simulink model "MIL4L3_SW6_V1_20220211"  (R2018b)
settings: Solver=FixedStepAuto  StartTime=0.0  StopTime=inf  FixedStep=0.001  RelTol=1e-3
PreLoadFcn:
  | A0_MILtest;
undefined symbols (not defined in the file or in its folder): Clb_ICADirect_LaneDisp_StateFive, Clb_ICADirect_LaneDisp_StateFour, Clb_ICADirect_LaneDisp_StateOne, Clb_ICADirect_LaneDisp_StateThree, Clb_ICADirect_LaneDisp_StateTwo, Clb_ICADirect_LaneDisp_StateZero, Clb_ICADirect_LaneDispSW, Clb_ICADirect_TrnLghtsCom_Switch, Clb_ICADirect_TrnLghtsCom_Value, Clb_ICADirect_TrnLghtsCrtl_Inhb, IMAP_Clb_ACU_Driver_Belt, IMAP_Clb_ACU_Driver_Belt_Over, IMAP_Clb_ACU_Passenger_Belt, IMAP_Clb_ACU_Passenger_Belt_Over, IMAP_Clb_ACU_RearLeft_Belt, IMAP_Clb_ACU_RearLeft_Belt_Over, IMAP_Clb_ACU_RearMiddle_Belt, IMAP_Clb_ACU_RearMiddle_Belt_Over, IMAP_Clb_ACU_RearRight_Belt, IMAP_Clb_ACU_RearRight_Belt_Over, IMAP_Clb_AEB_Switch, IMAP_Clb_AEB_Switch_Over, IMAP_Clb_ALC_TLC_Mode, IMAP_Clb_ALC_TLC_Mode_Over, IMAP_Clb_BCM_Battery_Voltage, IMAP_Clb_BCM_Battery_Voltage_Over, IMAP_Clb_BCM_BrakeLamp_State, IMAP_Clb_BCM_BrakeLamp_State_Over, IMAP_Clb_BCM_CHMSL_Status, IMAP_Clb_BCM_CHMSL_Status_Over, IMAP_Clb_BCM_Door_Lock_State, IMAP_Clb_BCM_Door_Lock_State_Over, IMAP_Clb_BCM_FrontWiper_State, IMAP_Clb_BCM_FrontWiper_State_Over, IMAP_Clb_BCM_FrontWiper_Switch, IMAP_Clb_BCM_FrontWiper_Switch_Over, IMAP_Clb_BCM_HazardLamp, IMAP_Clb_BCM_HazardLamp_Over, IMAP_Clb_BCM_HazardLamp_Switch, IMAP_Clb_BCM_HazardLamp_Switch_Over, IMAP_Clb_BCM_HighBeam_State, IMAP_Clb_BCM_HighBeam_State_Over, IMAP_Clb_BCM_Ignition_State, IMAP_Clb_BCM_Ignition_State_Over, IMAP_Clb_BCM_IHBC_Enabled, IMAP_Clb_BCM_IHBC_Enabled_Over, IMAP_Clb_BCM_Left_Light, IMAP_Clb_BCM_Left_Light_Over, IMAP_Clb_BCM_LeftTurn_Switch, IMAP_Clb_BCM_LeftTurn_Switch_Over, IMAP_Clb_BCM_LF_Door_State, IMAP_Clb_BCM_LF_Door_State_Over, IMAP_Clb_BCM_LowBeam_State, IMAP_Clb_BCM_LowBeam_State_Over, IMAP_Clb_BCM_LR_Door_State, IMAP_Clb_BCM_LR_Door_State_Over, IMAP_Clb_BCM_RF_Door_State, IMAP_Clb_BCM_RF_Door_State_Over, IMAP_Clb_BCM_Right_Light, IMAP_Clb_BCM_Right_Light_Over ... (+547)
libraries: CarMaker4SL x2153, simulink x292, dspstat3 x3, canmsglib x2, simulink_extras x1
(part 27 of 52)

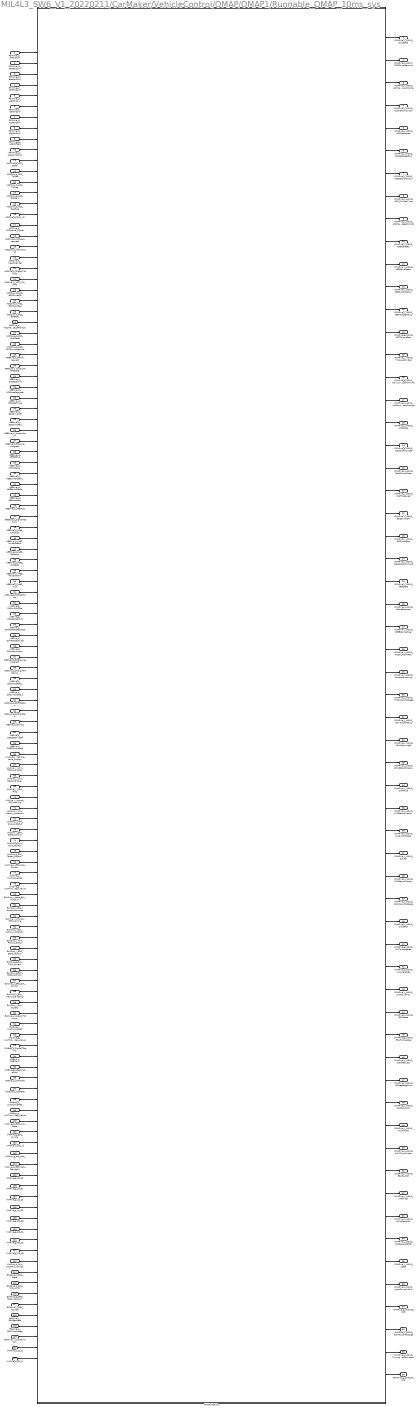
== system MIL4L3_SW6_V1_20220211/CarMaker/VehicleControl/OMAP/OMAP1/Runnable_OMAP_10ms_sys ==
  FDMMve_d_JaFcnConf : Inport  OutDataTypeStr=uint16  PortDimensions=1
  FDMMve_d_AebFcnConf : Inport  Port=2  OutDataTypeStr=uint16  PortDimensions=1
  FDMMve_d_EsaFcnConf : Inport  Port=3  OutDataTypeStr=uint16  PortDimensions=1
  FDMMve_d_ElkFcnConf : Inport  Port=4  OutDataTypeStr=uint16  PortDimensions=1
  FDMMve_d_LkaFcnConf : Inport  Port=5  OutDataTypeStr=uint16  PortDimensions=1
  FDMMve_d_IcaFcnConf : Inport  Port=6  OutDataTypeStr=uint16  PortDimensions=1
  FDMMve_d_AccFcnConf : Inport  Port=7  OutDataTypeStr=uint16  PortDimensions=1
  FDMMve_d_EwFcnConf : Inport  Port=8  OutDataTypeStr=uint16  PortDimensions=1
  FDMMve_g_Adas2Fapa : Inport  Port=9  OutDataTypeStr=uint32  PortDimensions=1
  FDMMve_d_SignalTStamp : Inport  Port=10  OutDataTypeStr=uint16  PortDimensions=1
  ACCSve_d_ACC_State : Inport  Port=11  OutDataTypeStr=uint16  PortDimensions=1
  ACCSve_g_ACC_TqReq : Inport  Port=12  OutDataTypeStr=single  PortDimensions=1
  ACCSve_d_ACC_TqFlag : Inport  Port=13  OutDataTypeStr=uint16  PortDimensions=1
  ACCSve_g_ACC_DecReq : Inport  Port=14  OutDataTypeStr=single  PortDimensions=1
  ACCSve_d_ACC_DecFlag : Inport  Port=15  OutDataTypeStr=uint16  PortDimensions=1
  ACCSve_d_CIPV_ID : Inport  Port=16  OutDataTypeStr=uint16  PortDimensions=1
  ACCSve_d_ACCActive_Signal : Inport  Port=17  OutDataTypeStr=uint16  PortDimensions=1
  ACCSve_d_ACC_go_request : Inport  Port=18  OutDataTypeStr=uint16  PortDimensions=1
  ACCSve_d_VelocitySet : Inport  Port=19  OutDataTypeStr=uint16  PortDimensions=1
  ACCSve_d_HeadWaySet : Inport  Port=20  OutDataTypeStr=uint16  PortDimensions=1
  ACCSve_d_SignalTStamp : Inport  Port=21  OutDataTypeStr=uint16  PortDimensions=1
  ACCSve_d_ACC_ICA_Flag : Inport  Port=22  OutDataTypeStr=uint16  PortDimensions=1
  ACCSve_d_ACC_ESCDriveOff : Inport  Port=23  OutDataTypeStr=uint16  PortDimensions=1
  ACCSve_d_ACC_ESCHoldReq : Inport  Port=24  OutDataTypeStr=uint16  PortDimensions=1
  ACCSve_d_ACC_EPBReq : Inport  Port=25  OutDataTypeStr=uint16  PortDimensions=1
  ACCSve_d_ACCMessagePrompt : Inport  Port=26  OutDataTypeStr=uint16
  ACCSve_d_ACC_ISLCState : Inport  Port=27  OutDataTypeStr=uint16  PortDimensions=1
  ACCSve_d_ACC_ISLCDriverRemind : Inport  Port=28  OutDataTypeStr=uint16  PortDimensions=1
  AEBSve_d_Prefill_request : Inport  Port=29  OutDataTypeStr=uint16  PortDimensions=1
  AEBSve_d_functionFARCState : Inport  Port=30  OutDataTypeStr=uint16  PortDimensions=1
  AEBSve_g_DecSetpoint : Inport  Port=31  OutDataTypeStr=single  PortDimensions=1
  AEBSve_d_MDDdecRequest : Inport  Port=32  OutDataTypeStr=uint16  PortDimensions=1
  AEBSve_d_MDDdecType : Inport  Port=33  OutDataTypeStr=uint16  PortDimensions=1
  AEBSve_d_ESCDriveOff : Inport  Port=34  OutDataTypeStr=uint16  PortDimensions=1
  AEBSve_d_ESCHoldReq : Inport  Port=35  OutDataTypeStr=uint16  PortDimensions=1
  AEBSve_d_HapticAlarm : Inport  Port=36  OutDataTypeStr=uint16  PortDimensions=1
  AEBSve_d_Braking_progress : Inport  Port=37  OutDataTypeStr=uint16  PortDimensions=1
  AEBSve_d_AEBStatus : Inport  Port=38  OutDataTypeStr=uint16  PortDimensions=1
  AEBSve_d_FCWStatus : Inport  Port=39  OutDataTypeStr=uint16  PortDimensions=1
  AEBSve_d_AEBSwitchStatus : Inport  Port=40  OutDataTypeStr=uint16  PortDimensions=1
  AEBSve_d_AEBFaultStatus : Inport  Port=41  OutDataTypeStr=uint16  PortDimensions=1
  AEBSve_d_AEBAlertReq : Inport  Port=42  OutDataTypeStr=uint16  PortDimensions=1
  AEBSve_d_AEBTips : Inport  Port=43  OutDataTypeStr=uint16  PortDimensions=1
  AEBSve_d_SignalTStamp : Inport  Port=44  OutDataTypeStr=uint16  PortDimensions=1
  AEBSve_d_JABS_AlertSign : Inport  Port=45  OutDataTypeStr=uint16  PortDimensions=1
  AEBSve_d_JABS_SwitchStatus : Inport  Port=46  OutDataTypeStr=uint16  PortDimensions=1
  AEBSve_d_JABS_FltStatus : Inport  Port=47  OutDataTypeStr=uint16  PortDimensions=1
  AEBSve_d_JABS_AlertReq : Inport  Port=48  OutDataTypeStr=uint16  PortDimensions=1
  AEBSve_d_JABS_HapticAlarm : Inport  Port=49  OutDataTypeStr=uint16  PortDimensions=1
  AEBSve_d_JABS_Tips : Inport  Port=50  OutDataTypeStr=uint16  PortDimensions=1
  JABSve_d_DbPrefillReq : Inport  Port=51  OutDataTypeStr=uint16  PortDimensions=1
  JABSve_d_DbFunFARCSta : Inport  Port=52  OutDataTypeStr=uint16  PortDimensions=1
  JABSve_g_DbDecSetpoint : Inport  Port=53  OutDataTypeStr=single  PortDimensions=1
  JABSve_d_DbMDDdecRequest : Inport  Port=54  OutDataTypeStr=uint16  PortDimensions=1
  JABSve_d_DbMDDdecType : Inport  Port=55  OutDataTypeStr=uint16  PortDimensions=1
  JABSve_d_DbHapticAlarm : Inport  Port=56  OutDataTypeStr=uint16  PortDimensions=1
  JABSve_d_DbBraking_progress : Inport  Port=57  OutDataTypeStr=uint16  PortDimensions=1
  JABSve_d_DbSignalTStamp : Inport  Port=58  OutDataTypeStr=uint16  PortDimensions=1
  JABSve_d_DbJACWStatus : Inport  Port=59  OutDataTypeStr=uint16  PortDimensions=1
  JABSve_d_DbSwitchStatus : Inport  Port=60  OutDataTypeStr=uint16  PortDimensions=1
  JABSve_d_DbFltStatus : Inport  Port=61  OutDataTypeStr=uint16  PortDimensions=1
  JABSve_d_DbAlertReq : Inport  Port=62  OutDataTypeStr=uint16  PortDimensions=1
  JABSve_d_DbTips : Inport  Port=63  OutDataTypeStr=uint16  PortDimensions=1
  JABSve_d_DbESCDriveOff : Inport  Port=64  OutDataTypeStr=uint16  PortDimensions=1
  JABSve_d_DbESCHoldReq : Inport  Port=65  OutDataTypeStr=uint16  PortDimensions=1
  LKASve_y_Vehicle_Lane_Display : Inport  Port=66  OutDataTypeStr=uint8  PortDimensions=1
  LKASve_y_LDW_Status_Display : Inport  Port=67  OutDataTypeStr=uint8  PortDimensions=1
  LKASve_y_LKA_Status_Display : Inport  Port=68  OutDataTypeStr=uint8  PortDimensions=1
  LKASve_y_LDW_Flag : Inport  Port=69  OutDataTypeStr=uint8  PortDimensions=1
  LKASve_y_Hands_Off_Warning : Inport  Port=70  OutDataTypeStr=uint8  PortDimensions=1
  LKASve_y_LKA_Action_Indication : Inport  Port=71  OutDataTypeStr=uint8  PortDimensions=1
  LKASve_y_HMI_Popup_Status : Inport  Port=72  OutDataTypeStr=uint8  PortDimensions=1
  LKASve_y_EPS_State_Control : Inport  Port=73  OutDataTypeStr=uint8  PortDimensions=1
  LKASve_g_LKA_SWA_Control : Inport  Port=74  OutDataTypeStr=single  PortDimensions=1
  LKASve_g_EPS_Factor_Control : Inport  Port=75  OutDataTypeStr=single  PortDimensions=1
  LKASve_y_EPS_LKA_Control : Inport  Port=76  OutDataTypeStr=uint8  PortDimensions=1
  LKASve_y_LKATorqueReq : Inport  Port=77  OutDataTypeStr=uint8  PortDimensions=1
  LKASve_g_LKATorqueReq_Value : Inport  Port=78  OutDataTypeStr=single  PortDimensions=1
  ELKSve_y_state_ELK_function : Inport  Port=79  OutDataTypeStr=uint8  PortDimensions=1
  ELKSve_y_ELK_HapticAlarmReq : Inport  Port=80  OutDataTypeStr=uint8  PortDimensions=1
  ELKSve_y_Hands_Off_Warning : Inport  Port=81  OutDataTypeStr=uint8  PortDimensions=1
  ELKSve_y_ELK_Action_Indication : Inport  Port=82  OutDataTypeStr=uint8  PortDimensions=1
  ELKSve_y_HMI_Popup_Status : Inport  Port=83  OutDataTypeStr=uint8  PortDimensions=1
  ELKSve_y_EPS_State_Control : Inport  Port=84  OutDataTypeStr=uint8  PortDimensions=1
  ELKSve_g_ELK_SWA_Control : Inport  Port=85  OutDataTypeStr=single  PortDimensions=1
  ELKSve_g_EPS_Factor_Control : Inport  Port=86  OutDataTypeStr=single  PortDimensions=1
  ELKSve_y_EPS_ELK_Control : Inport  Port=87  OutDataTypeStr=uint8  PortDimensions=1
  ELKSve_y_ELK_VehicleLaneDisp : Inport  Port=88  OutDataTypeStr=uint8  PortDimensions=1
  ELKSve_y_ELK_ELKSts : Inport  Port=89  OutDataTypeStr=uint8  PortDimensions=1
  ELKSve_y_SignalTStamp : Inport  Port=90  OutDataTypeStr=uint8  PortDimensions=1
  ELKSve_y_LKATorqueReq : Inport  Port=91  OutDataTypeStr=uint8  PortDimensions=1
  ELKSve_g_LKATorqueReq_Value : Inport  Port=92  OutDataTypeStr=single  PortDimensions=1
  ICABve_d_SignalTStamp : Inport  Port=93  OutDataTypeStr=uint16  PortDimensions=1
  ICABva_d_ICAB2HMI : Inport  Port=94  OutDataTypeStr=uint16  PortDimensions=20
  ICABve_g_SteerAngleCmd : Inport  Port=95  OutDataTypeStr=single  PortDimensions=1
  ICABve_d_ICAMode : Inport  Port=96  OutDataTypeStr=uint16  PortDimensions=1
  ICABve_d_ICAState : Inport  Port=97  OutDataTypeStr=uint16  PortDimensions=1
  ICABve_d_LKATorqueReq : Inport  Port=98  OutDataTypeStr=uint16  PortDimensions=1
  ICABve_g_LKATorqueReq_Value : Inport  Port=99  OutDataTypeStr=single  PortDimensions=1
  IMAPve_d_EPS_LKA_State : Inport  Port=100  OutDataTypeStr=uint16  PortDimensions=1
  IMAPve_g_ESC_LonAcc : Inport  Port=101  OutDataTypeStr=single  PortDimensions=1
  IMAPva_d_obj_id : Inport  Port=102  OutDataTypeStr=uint16  PortDimensions=40
  IMAPva_g_obj_pos_x : Inport  Port=103  OutDataTypeStr=single  PortDimensions=40
  IMAPve_d_ESC_Veh_Standstill : Inport  Port=104  OutDataTypeStr=uint16  PortDimensions=1
  IMAPve_g_L0_C0 : Inport  Port=105  OutDataTypeStr=single  PortDimensions=1
  IMAPve_g_L0_C1 : Inport  Port=106  OutDataTypeStr=single  PortDimensions=1
  IMAPve_g_L0_C2 : Inport  Port=107  OutDataTypeStr=single  PortDimensions=1
  IMAPve_g_L0_C3 : Inport  Port=108  OutDataTypeStr=single  PortDimensions=1
  IMAPve_g_R0_C0 : Inport  Port=109  OutDataTypeStr=single  PortDimensions=1
  IMAPve_g_R0_C1 : Inport  Port=110  OutDataTypeStr=single  PortDimensions=1
  IMAPve_g_R0_C2 : Inport  Port=111  OutDataTypeStr=single  PortDimensions=1
  IMAPve_g_R0_C3 : Inport  Port=112  OutDataTypeStr=single  PortDimensions=1
  IMAPve_d_APA_AutoPark_WorkSt : Inport  Port=113  OutDataTypeStr=uint16  PortDimensions=1
  ESASve_y_ESA_State : Inport  Port=114  OutDataTypeStr=uint8
  ESASve_g_ESA_SWA_CMD : Inport  Port=115  OutDataTypeStr=single
  ESASve_g_EPS_Factor_Control : Inport  Port=116  OutDataTypeStr=single
  ESASve_y_ESA_FaultSt : Inport  Port=117  OutDataTypeStr=uint8
  ESASve_y_ESARequest : Inport  Port=118  OutDataTypeStr=uint8
  ESASve_y_ESATorqueReq : Inport  Port=119  OutDataTypeStr=single
  ESASve_y_LKAActivation : Inport  Port=120  OutDataTypeStr=uint8
  IMAPve_d_L0_Q : Inport  Port=121  OutDataTypeStr=uint16
  IMAPve_d_R0_Q : Inport  Port=122  OutDataTypeStr=uint16
  OMAP_Module : Subsystem  TreatAsAtomicUnit=on
  OMAPve_y_ADAS_ISLCState : Outport  OutDataTypeStr=uint8  PortDimensions=1
  OMAPve_y_ADAS_ISLCDriverRemind : Outport  Port=2  OutDataTypeStr=uint8  PortDimensions=1
  OMAPve_y_ADAS_ACCHeadwayDisplay : Outport  Port=3  OutDataTypeStr=uint8  PortDimensions=1
  OMAPve_y_ADAS_ACCHeadwayIcon : Outport  Port=4  OutDataTypeStr=uint8  PortDimensions=1
  OMAPve_y_ADAS_ACCSetSpeed : Outport  Port=5  OutDataTypeStr=uint8  PortDimensions=1
  OMAPve_y_ADAS_ACCSetSpeedDis : Outport  Port=6  OutDataTypeStr=uint8  PortDimensions=1
  OMAPve_y_ADAS_ACCStatusIconDis : Outport  Port=7  OutDataTypeStr=uint8  PortDimensions=1
  OMAPve_y_ADAS_ACC_RVVReqType : Outport  Port=8  OutDataTypeStr=uint8  PortDimensions=1
  OMAPve_y_ADAS_ACCMessagePrompt : Outport  Port=9  OutDataTypeStr=uint8  PortDimensions=1
  OMAPve_y_ADAS_AEBAlertReq : Outport  Port=10  OutDataTypeStr=uint8  PortDimensions=1
  OMAPve_y_ADAS_AEBFaultStatus : Outport  Port=11  OutDataTypeStr=uint8  PortDimensions=1
  OMAPve_y_ADAS_AEBSwitchStatus : Outport  Port=12  OutDataTypeStr=uint8  PortDimensions=1
  OMAPve_y_ADAS_AEBMassageDisp : Outport  Port=13  OutDataTypeStr=uint8  PortDimensions=1
  OMAPve_g_ADAS_ACCTorqueReq : Outport  Port=14  OutDataTypeStr=single  PortDimensions=1
  OMAPve_y_ADAS_TorqueActivReq : Outport  Port=15  OutDataTypeStr=uint8  PortDimensions=1
  OMAPve_g_ADAS_DownorUpGearMinTime : Outport  Port=16  OutDataTypeStr=single  PortDimensions=1
  OMAPve_y_ADAS_UpDownGearChange : Outport  Port=17  OutDataTypeStr=uint8  PortDimensions=1
  OMAPve_y_ADAS_ACCState : Outport  Port=18  OutDataTypeStr=uint8  PortDimensions=1
  OMAPve_g_ADAS_DecelerationSet : Outport  Port=19  OutDataTypeStr=single  PortDimensions=1
  OMAPve_y_ADAS_DeclControlReq : Outport  Port=20  OutDataTypeStr=uint8  PortDimensions=1
  OMAPve_y_ADAS_PrefillRequest : Outport  Port=21  OutDataTypeStr=uint8  PortDimensions=1
  OMAPve_y_ADAS_ESCDriveOff : Outport  Port=22  OutDataTypeStr=uint8  PortDimensions=1
  OMAPve_y_ADAS_ESCHoldReq : Outport  Port=23  OutDataTypeStr=uint8  PortDimensions=1
  OMAPve_y_ADAS_DecelerationType : Outport  Port=24  OutDataTypeStr=uint8  PortDimensions=1
  OMAPve_y_ADAS_AEBState : Outport  Port=25  OutDataTypeStr=uint8  PortDimensions=1
  OMAPve_y_ADAS_BrakeRequest : Outport  Port=26  OutDataTypeStr=uint8  PortDimensions=1
  OMAPve_y_ADAS_AEBBrakingProg : Outport  Port=27  OutDataTypeStr=uint8  PortDimensions=1
  OMAPve_y_ADAS_HapticAlarmReq : Outport  Port=28  OutDataTypeStr=uint8  PortDimensions=1
  OMAPve_y_ADAS_Handsoffwarning : Outport  Port=29  OutDataTypeStr=uint8  PortDimensions=1
  OMAPve_y_ADAS_HMIPopupMassage : Outport  Port=30  OutDataTypeStr=uint8  PortDimensions=1
  OMAPve_y_ADAS_VehicleLaneDisp : Outport  Port=31  OutDataTypeStr=uint8  PortDimensions=1
  OMAPve_y_ADAS_LDWWarningSt : Outport  Port=32  OutDataTypeStr=uint8  PortDimensions=1
  OMAPve_y_ADAS_LDWStatusDisplay : Outport  Port=33  OutDataTypeStr=uint8  PortDimensions=1
  OMAPve_y_ADAS_LKAMode : Outport  Port=34  OutDataTypeStr=uint8  PortDimensions=1
  OMAPve_y_ADAS_LKAStatusDisplay : Outport  Port=35  OutDataTypeStr=uint8  PortDimensions=1
  OMAPve_y_ADAS_LKASwitchState : Outport  Port=36  OutDataTypeStr=uint8  PortDimensions=1
  OMAPve_y_ADAS_ELKSts : Outport  Port=37  OutDataTypeStr=uint8  PortDimensions=1
  OMAPve_y_ADAS_LCAStatusDisplay : Outport  Port=38  OutDataTypeStr=uint8  PortDimensions=1
  OMAPve_y_ADAS_LCAPopupMessage : Outport  Port=39  OutDataTypeStr=uint8  PortDimensions=1
  OMAPve_y_ADAS_LKAState : Outport  Port=40  OutDataTypeStr=uint8  PortDimensions=1
  OMAPve_g_ADAS_LKATorqFactReq : Outport  Port=41  OutDataTypeStr=single  PortDimensions=1
  OMAPve_g_ADAS_LKAAngleReq : Outport  Port=42  OutDataTypeStr=single  PortDimensions=1
  OMAPve_y_ADAS_LKAActivation : Outport  Port=43  OutDataTypeStr=uint8  PortDimensions=1
  OMAPve_y_ADAS_ESAState : Outport  Port=44  OutDataTypeStr=uint8  PortDimensions=1
  OMAPve_g_ADAS_ESATorqueReq : Outport  Port=45  OutDataTypeStr=single  PortDimensions=1
  OMAPve_y_ADAS_ESARequest : Outport  Port=46  OutDataTypeStr=uint8  PortDimensions=1
  OMAPve_y_ADAS_ICAMassageDisp : Outport  Port=47  OutDataTypeStr=uint8  PortDimensions=1
  OMAPve_y_ADAS_ICAStatusIcon : Outport  Port=48  OutDataTypeStr=uint8  PortDimensions=1
  OMAPve_y_ADAS_HWAMode : Outport  Port=49  OutDataTypeStr=uint8  PortDimensions=1
  OMAPve_y_ADAS_HWATurnOnIdctr : Outport  Port=50  OutDataTypeStr=uint8  PortDimensions=1
  OMAPve_y_ADAS_ESAFaultSt : Outport  Port=51  OutDataTypeStr=uint8  PortDimensions=1
  OMAPve_y_ADAS_JAFaultSt : Outport  Port=52  OutDataTypeStr=uint8  PortDimensions=1
  OMAPve_y_ADAS_HWAActionSts : Outport  Port=53  OutDataTypeStr=uint8  PortDimensions=1
  OMAPve_y_ADAS_ACCRequestEPB : Outport  Port=54  OutDataTypeStr=uint8  PortDimensions=1
  OMAPve_y_ADAS_State : Outport  Port=55  OutDataTypeStr=uint8  PortDimensions=1
  OMAPve_y_ADAS_LightControlValid : Outport  Port=56  OutDataTypeStr=uint8  PortDimensions=1
  OMAPve_g_ob019L_100 : Outport  Port=57  OutDataTypeStr=uint32  PortDimensions=1
  OMAPve_y_ADAS_ELKPopupMessage : Outport  Port=58  OutDataTypeStr=uint8
  OMAPve_y_ADAS_TurnLightsCommand : Outport  Port=59  OutDataTypeStr=uint8
  FDMMve_g_ob019H_100 : Outport  Port=60  OutDataTypeStr=uint32
  wires:
  ELKSve_y_HMI_Popup_Status/1 -> OMAP_Module/83(ELKSve_y_HMI_Popup_Status)
  FDMMve_d_ElkFcnConf/1 -> OMAP_Module/4(FDMMve_d_ElkFcnConf)
  AEBSve_d_AEBFaultStatus/1 -> OMAP_Module/41(AEBSve_d_AEBFaultStatus)
  OMAP_Module/36(OMAPve_y_ADAS_LKASwitchState) -> OMAPve_y_ADAS_LKASwitchState/1
  AEBSve_d_Braking_progress/1 -> OMAP_Module/37(AEBSve_d_Braking_progress)
  OMAP_Module/9(OMAPve_y_ADAS_ACCMessagePrompt) -> OMAPve_y_ADAS_ACCMessagePrompt/1
  OMAP_Module/31(OMAPve_y_ADAS_VehicleLaneDisp) -> OMAPve_y_ADAS_VehicleLaneDisp/1
  FDMMve_d_AebFcnConf/1 -> OMAP_Module/2(FDMMve_d_AebFcnConf)
  ACCSve_d_ACC_DecFlag/1 -> OMAP_Module/15(ACCSve_d_ACC_DecFlag)
  ICABva_d_ICAB2HMI/1 -> OMAP_Module/94(ICABva_d_ICAB2HMI)
  OMAP_Module/32(OMAPve_y_ADAS_LDWWarningSt) -> OMAPve_y_ADAS_LDWWarningSt/1
  AEBSve_d_AEBStatus/1 -> OMAP_Module/38(AEBSve_d_AEBStatus)
  IMAPve_d_ESC_Veh_Standstill/1 -> OMAP_Module/104(IMAPve_d_ESC_Veh_Standstill)
  FDMMve_g_Adas2Fapa/1 -> OMAP_Module/9(FDMMve_g_Adas2Fapa)
  OMAP_Module/41(OMAPve_g_ADAS_LKATorqFactReq) -> OMAPve_g_ADAS_LKATorqFactReq/1
  ELKSve_g_ELK_SWA_Control/1 -> OMAP_Module/85(ELKSve_g_ELK_SWA_Control)
  FDMMve_d_IcaFcnConf/1 -> OMAP_Module/6(FDMMve_d_IcaFcnConf)
  LKASve_y_EPS_State_Control/1 -> OMAP_Module/73(LKASve_y_EPS_State_Control)
  OMAP_Module/14(OMAPve_g_ADAS_ACCTorqueReq) -> OMAPve_g_ADAS_ACCTorqueReq/1
  ELKSve_y_ELK_ELKSts/1 -> OMAP_Module/89(ELKSve_y_ELK_ELKSts)
  ICABve_d_SignalTStamp/1 -> OMAP_Module/93(ICABve_d_SignalTStamp)
  AEBSve_d_MDDdecRequest/1 -> OMAP_Module/32(AEBSve_d_MDDdecRequest)
  ELKSve_y_state_ELK_function/1 -> OMAP_Module/79(ELKSve_y_state_ELK_function)
  OMAP_Module/6(OMAPve_y_ADAS_ACCSetSpeedDis) -> OMAPve_y_ADAS_ACCSetSpeedDis/1
  ACCSve_d_ACCActive_Signal/1 -> OMAP_Module/17(ACCSve_d_ACCActive_Signal)
  AEBSve_g_DecSetpoint/1 -> OMAP_Module/31(AEBSve_g_DecSetpoint)
  IMAPve_g_L0_C2/1 -> OMAP_Module/107(IMAPve_g_L0_C2)
  JABSve_d_DbSwitchStatus/1 -> OMAP_Module/60(JABSve_d_DbSwitchStatus)
  ACCSve_d_VelocitySet/1 -> OMAP_Module/19(ACCSve_d_VelocitySet)
  ELKSve_y_SignalTStamp/1 -> OMAP_Module/90(ELKSve_y_SignalTStamp)
  ACCSve_d_ACC_ICA_Flag/1 -> OMAP_Module/22(ACCSve_d_ACC_ICA_Flag)
  AEBSve_d_AEBAlertReq/1 -> OMAP_Module/42(AEBSve_d_AEBAlertReq)
  JABSve_d_DbMDDdecType/1 -> OMAP_Module/55(JABSve_d_DbMDDdecType)
  OMAP_Module/13(OMAPve_y_ADAS_AEBMassageDisp) -> OMAPve_y_ADAS_AEBMassageDisp/1
  LKASve_y_EPS_LKA_Control/1 -> OMAP_Module/76(LKASve_y_EPS_LKA_Control)
  ELKSve_y_ELK_Action_Indication/1 -> OMAP_Module/82(ELKSve_y_ELK_Action_Indication)
  AEBSve_d_JABS_FltStatus/1 -> OMAP_Module/47(AEBSve_d_JABS_FltStatus)
  OMAP_Module/47(OMAPve_y_ADAS_ICAMassageDisp) -> OMAPve_y_ADAS_ICAMassageDisp/1
  OMAP_Module/4(OMAPve_y_ADAS_ACCHeadwayIcon) -> OMAPve_y_ADAS_ACCHeadwayIcon/1
  OMAP_Module/8(OMAPve_y_ADAS_ACC_RVVReqType) -> OMAPve_y_ADAS_ACC_RVVReqType/1
  JABSve_d_DbPrefillReq/1 -> OMAP_Module/51(JABSve_d_DbPrefillReq)
  LKASve_y_LDW_Status_Display/1 -> OMAP_Module/67(LKASve_y_LDW_Status_Display)
  AEBSve_d_JABS_Tips/1 -> OMAP_Module/50(AEBSve_d_JABS_Tips)
  AEBSve_d_JABS_AlertReq/1 -> OMAP_Module/48(AEBSve_d_JABS_AlertReq)
  AEBSve_d_JABS_AlertSign/1 -> OMAP_Module/45(AEBSve_d_JABS_AlertSign)
  OMAP_Module/11(OMAPve_y_ADAS_AEBFaultStatus) -> OMAPve_y_ADAS_AEBFaultStatus/1
  AEBSve_d_FCWStatus/1 -> OMAP_Module/39(AEBSve_d_FCWStatus)
  JABSve_d_DbFunFARCSta/1 -> OMAP_Module/52(JABSve_d_DbFunFARCSta)
  AEBSve_d_SignalTStamp/1 -> OMAP_Module/44(AEBSve_d_SignalTStamp)
  ELKSve_g_EPS_Factor_Control/1 -> OMAP_Module/86(ELKSve_g_EPS_Factor_Control)
  IMAPve_g_R0_C1/1 -> OMAP_Module/110(IMAPve_g_R0_C1)
  JABSve_d_DbTips/1 -> OMAP_Module/63(JABSve_d_DbTips)
  AEBSve_d_functionFARCState/1 -> OMAP_Module/30(AEBSve_d_functionFARCState)
  JABSve_d_DbBraking_progress/1 -> OMAP_Module/57(JABSve_d_DbBraking_progress)
  AEBSve_d_MDDdecType/1 -> OMAP_Module/33(AEBSve_d_MDDdecType)
  LKASve_y_Vehicle_Lane_Display/1 -> OMAP_Module/66(LKASve_y_Vehicle_Lane_Display)
  AEBSve_d_HapticAlarm/1 -> OMAP_Module/36(AEBSve_d_HapticAlarm)
  OMAP_Module/12(OMAPve_y_ADAS_AEBSwitchStatus) -> OMAPve_y_ADAS_AEBSwitchStatus/1
  OMAP_Module/5(OMAPve_y_ADAS_ACCSetSpeed) -> OMAPve_y_ADAS_ACCSetSpeed/1
  ELKSve_y_EPS_State_Control/1 -> OMAP_Module/84(ELKSve_y_EPS_State_Control)
  OMAP_Module/26(OMAPve_y_ADAS_BrakeRequest) -> OMAPve_y_ADAS_BrakeRequest/1
  AEBSve_d_ESCHoldReq/1 -> OMAP_Module/35(AEBSve_d_ESCHoldReq)
  OMAP_Module/21(OMAPve_y_ADAS_PrefillRequest) -> OMAPve_y_ADAS_PrefillRequest/1
  OMAP_Module/43(OMAPve_y_ADAS_LKAActivation) -> OMAPve_y_ADAS_LKAActivation/1
  ACCSve_g_ACC_DecReq/1 -> OMAP_Module/14(ACCSve_g_ACC_DecReq)
  ACCSve_g_ACC_TqReq/1 -> OMAP_Module/12(ACCSve_g_ACC_TqReq)
  OMAP_Module/10(OMAPve_y_ADAS_AEBAlertReq) -> OMAPve_y_ADAS_AEBAlertReq/1
  OMAP_Module/50(OMAPve_y_ADAS_HWATurnOnIdctr) -> OMAPve_y_ADAS_HWATurnOnIdctr/1
  JABSve_d_DbSignalTStamp/1 -> OMAP_Module/58(JABSve_d_DbSignalTStamp)
  ELKSve_y_EPS_ELK_Control/1 -> OMAP_Module/87(ELKSve_y_EPS_ELK_Control)
  IMAPve_g_L0_C0/1 -> OMAP_Module/105(IMAPve_g_L0_C0)
  IMAPva_d_obj_id/1 -> OMAP_Module/102(IMAPva_d_obj_id)
  OMAP_Module/2(OMAPve_y_ADAS_ISLCDriverRemind) -> OMAPve_y_ADAS_ISLCDriverRemind/1
  JABSve_d_DbHapticAlarm/1 -> OMAP_Module/56(JABSve_d_DbHapticAlarm)
  AEBSve_d_AEBTips/1 -> OMAP_Module/43(AEBSve_d_AEBTips)
  IMAPve_g_R0_C3/1 -> OMAP_Module/112(IMAPve_g_R0_C3)
  ACCSve_d_CIPV_ID/1 -> OMAP_Module/16(ACCSve_d_CIPV_ID)
  OMAP_Module/27(OMAPve_y_ADAS_AEBBrakingProg) -> OMAPve_y_ADAS_AEBBrakingProg/1
  LKASve_y_LKA_Action_Indication/1 -> OMAP_Module/71(LKASve_y_LKA_Action_Indication)
  OMAP_Module/3(OMAPve_y_ADAS_ACCHeadwayDisplay) -> OMAPve_y_ADAS_ACCHeadwayDisplay/1
  ACCSve_d_ACC_go_request/1 -> OMAP_Module/18(ACCSve_d_ACC_go_request)
  IMAPve_g_L0_C1/1 -> OMAP_Module/106(IMAPve_g_L0_C1)
  LKASve_g_EPS_Factor_Control/1 -> OMAP_Module/75(LKASve_g_EPS_Factor_Control)
  OMAP_Module/22(OMAPve_y_ADAS_ESCDriveOff) -> OMAPve_y_ADAS_ESCDriveOff/1
  JABSve_d_DbMDDdecRequest/1 -> OMAP_Module/54(JABSve_d_DbMDDdecRequest)
  OMAP_Module/38(OMAPve_y_ADAS_LCAStatusDisplay) -> OMAPve_y_ADAS_LCAStatusDisplay/1
  OMAP_Module/28(OMAPve_y_ADAS_HapticAlarmReq) -> OMAPve_y_ADAS_HapticAlarmReq/1
  FDMMve_d_AccFcnConf/1 -> OMAP_Module/7(FDMMve_d_AccFcnConf)
  JABSve_d_DbESCHoldReq/1 -> OMAP_Module/65(JABSve_d_DbESCHoldReq)
  OMAP_Module/25(OMAPve_y_ADAS_AEBState) -> OMAPve_y_ADAS_AEBState/1
  OMAP_Module/16(OMAPve_g_ADAS_DownorUpGearMinTime) -> OMAPve_g_ADAS_DownorUpGearMinTime/1
  OMAP_Module/20(OMAPve_y_ADAS_DeclControlReq) -> OMAPve_y_ADAS_DeclControlReq/1
  OMAP_Module/29(OMAPve_y_ADAS_Handsoffwarning) -> OMAPve_y_ADAS_Handsoffwarning/1
  OMAP_Module/53(OMAPve_y_ADAS_HWAActionSts) -> OMAPve_y_ADAS_HWAActionSts/1
  OMAP_Module/15(OMAPve_y_ADAS_TorqueActivReq) -> OMAPve_y_ADAS_TorqueActivReq/1
  OMAP_Module/30(OMAPve_y_ADAS_HMIPopupMassage) -> OMAPve_y_ADAS_HMIPopupMassage/1
  IMAPve_g_ESC_LonAcc/1 -> OMAP_Module/101(IMAPve_g_ESC_LonAcc)
  AEBSve_d_Prefill_request/1 -> OMAP_Module/29(AEBSve_d_Prefill_request)
  ACCSve_d_ACC_ESCDriveOff/1 -> OMAP_Module/23(ACCSve_d_ACC_ESCDriveOff)
  IMAPve_g_R0_C0/1 -> OMAP_Module/109(IMAPve_g_R0_C0)
  OMAP_Module/34(OMAPve_y_ADAS_LKAMode) -> OMAPve_y_ADAS_LKAMode/1
  OMAP_Module/44(OMAPve_y_ADAS_ESAState) -> OMAPve_y_ADAS_ESAState/1
  OMAP_Module/33(OMAPve_y_ADAS_LDWStatusDisplay) -> OMAPve_y_ADAS_LDWStatusDisplay/1
  LKASve_y_LDW_Flag/1 -> OMAP_Module/69(LKASve_y_LDW_Flag)
  ELKSve_y_ELK_VehicleLaneDisp/1 -> OMAP_Module/88(ELKSve_y_ELK_VehicleLaneDisp)
  OMAP_Module/18(OMAPve_y_ADAS_ACCState) -> OMAPve_y_ADAS_ACCState/1
  OMAP_Module/52(OMAPve_y_ADAS_JAFaultSt) -> OMAPve_y_ADAS_JAFaultSt/1
  JABSve_d_DbFltStatus/1 -> OMAP_Module/61(JABSve_d_DbFltStatus)
  OMAP_Module/56(OMAPve_y_ADAS_LightControlValid) -> OMAPve_y_ADAS_LightControlValid/1
  ACCSve_d_ACC_ESCHoldReq/1 -> OMAP_Module/24(ACCSve_d_ACC_ESCHoldReq)
  OMAP_Module/54(OMAPve_y_ADAS_ACCRequestEPB) -> OMAPve_y_ADAS_ACCRequestEPB/1
  OMAP_Module/37(OMAPve_y_ADAS_ELKSts) -> OMAPve_y_ADAS_ELKSts/1
  LKASve_y_HMI_Popup_Status/1 -> OMAP_Module/72(LKASve_y_HMI_Popup_Status)
  OMAP_Module/7(OMAPve_y_ADAS_ACCStatusIconDis) -> OMAPve_y_ADAS_ACCStatusIconDis/1
  FDMMve_d_EwFcnConf/1 -> OMAP_Module/8(FDMMve_d_EwFcnConf)
  JABSve_d_DbJACWStatus/1 -> OMAP_Module/59(JABSve_d_DbJACWStatus)
  JABSve_g_DbDecSetpoint/1 -> OMAP_Module/53(JABSve_g_DbDecSetpoint)
  ICABve_d_ICAMode/1 -> OMAP_Module/96(ICABve_d_ICAMode)
  LKASve_y_Hands_Off_Warning/1 -> OMAP_Module/70(LKASve_y_Hands_Off_Warning)
  LKASve_y_LKA_Status_Display/1 -> OMAP_Module/68(LKASve_y_LKA_Status_Display)
  JABSve_d_DbAlertReq/1 -> OMAP_Module/62(JABSve_d_DbAlertReq)
  OMAP_Module/42(OMAPve_g_ADAS_LKAAngleReq) -> OMAPve_g_ADAS_LKAAngleReq/1
  OMAP_Module/40(OMAPve_y_ADAS_LKAState) -> OMAPve_y_ADAS_LKAState/1
  OMAP_Module/23(OMAPve_y_ADAS_ESCHoldReq) -> OMAPve_y_ADAS_ESCHoldReq/1
  AEBSve_d_JABS_HapticAlarm/1 -> OMAP_Module/49(AEBSve_d_JABS_HapticAlarm)
  OMAP_Module/45(OMAPve_g_ADAS_ESATorqueReq) -> OMAPve_g_ADAS_ESATorqueReq/1
  OMAP_Module/48(OMAPve_y_ADAS_ICAStatusIcon) -> OMAPve_y_ADAS_ICAStatusIcon/1
  OMAP_Module/17(OMAPve_y_ADAS_UpDownGearChange) -> OMAPve_y_ADAS_UpDownGearChange/1
  IMAPve_d_EPS_LKA_State/1 -> OMAP_Module/100(IMAPve_d_EPS_LKA_State)
  ACCSve_d_ACC_TqFlag/1 -> OMAP_Module/13(ACCSve_d_ACC_TqFlag)
  OMAP_Module/49(OMAPve_y_ADAS_HWAMode) -> OMAPve_y_ADAS_HWAMode/1
  FDMMve_d_EsaFcnConf/1 -> OMAP_Module/3(FDMMve_d_EsaFcnConf)
  IMAPve_g_R0_C2/1 -> OMAP_Module/111(IMAPve_g_R0_C2)
  OMAP_Module/24(OMAPve_y_ADAS_DecelerationType) -> OMAPve_y_ADAS_DecelerationType/1
  ACCSve_d_ACC_EPBReq/1 -> OMAP_Module/25(ACCSve_d_ACC_EPBReq)
  OMAP_Module/19(OMAPve_g_ADAS_DecelerationSet) -> OMAPve_g_ADAS_DecelerationSet/1
  AEBSve_d_AEBSwitchStatus/1 -> OMAP_Module/40(AEBSve_d_AEBSwitchStatus)
  JABSve_d_DbESCDriveOff/1 -> OMAP_Module/64(JABSve_d_DbESCDriveOff)
  OMAP_Module/35(OMAPve_y_ADAS_LKAStatusDisplay) -> OMAPve_y_ADAS_LKAStatusDisplay/1
  AEBSve_d_JABS_SwitchStatus/1 -> OMAP_Module/46(AEBSve_d_JABS_SwitchStatus)
  OMAP_Module/55(OMAPve_y_ADAS_State) -> OMAPve_y_ADAS_State/1
  OMAP_Module/51(OMAPve_y_ADAS_ESAFaultSt) -> OMAPve_y_ADAS_ESAFaultSt/1
  IMAPva_g_obj_pos_x/1 -> OMAP_Module/103(IMAPva_g_obj_pos_x)
  OMAP_Module/1(OMAPve_y_ADAS_ISLCState) -> OMAPve_y_ADAS_ISLCState/1
  ACCSve_d_SignalTStamp/1 -> OMAP_Module/21(ACCSve_d_SignalTStamp)
  FDMMve_d_LkaFcnConf/1 -> OMAP_Module/5(FDMMve_d_LkaFcnConf)
  OMAP_Module/46(OMAPve_y_ADAS_ESARequest) -> OMAPve_y_ADAS_ESARequest/1
  OMAP_Module/39(OMAPve_y_ADAS_LCAPopupMessage) -> OMAPve_y_ADAS_LCAPopupMessage/1
  ICABve_d_ICAState/1 -> OMAP_Module/97(ICABve_d_ICAState)
  ELKSve_y_Hands_Off_Warning/1 -> OMAP_Module/81(ELKSve_y_Hands_Off_Warning)
  AEBSve_d_ESCDriveOff/1 -> OMAP_Module/34(AEBSve_d_ESCDriveOff)
  ELKSve_y_ELK_HapticAlarmReq/1 -> OMAP_Module/80(ELKSve_y_ELK_HapticAlarmReq)
  ACCSve_d_HeadWaySet/1 -> OMAP_Module/20(ACCSve_d_HeadWaySet)
  LKASve_g_LKA_SWA_Control/1 -> OMAP_Module/74(LKASve_g_LKA_SWA_Control)
  ICABve_g_SteerAngleCmd/1 -> OMAP_Module/95(ICABve_g_SteerAngleCmd)
  IMAPve_g_L0_C3/1 -> OMAP_Module/108(IMAPve_g_L0_C3)
  FDMMve_d_JaFcnConf/1 -> OMAP_Module/1(FDMMve_d_JaFcnConf)
  FDMMve_d_SignalTStamp/1 -> OMAP_Module/10(FDMMve_d_SignalTStamp)
  ACCSve_d_ACC_State/1 -> OMAP_Module/11(ACCSve_d_ACC_State)
  LKASve_y_LKATorqueReq/1 -> OMAP_Module/77(LKASve_y_LKATorqueReq)
  LKASve_g_LKATorqueReq_Value/1 -> OMAP_Module/78(LKASve_g_LKATorqueReq_Value)
  ELKSve_y_LKATorqueReq/1 -> OMAP_Module/91(ELKSve_y_LKATorqueReq)
  ELKSve_g_LKATorqueReq_Value/1 -> OMAP_Module/92(ELKSve_g_LKATorqueReq_Value)
  ICABve_d_LKATorqueReq/1 -> OMAP_Module/98(ICABve_d_LKATorqueReq)
  ICABve_g_LKATorqueReq_Value/1 -> OMAP_Module/99(ICABve_g_LKATorqueReq_Value)
  IMAPve_d_APA_AutoPark_WorkSt/1 -> OMAP_Module/113(IMAPve_d_APA_AutoPark_WorkSt)
  OMAP_Module/57(OMAPve_g_ob019L_100) -> OMAPve_g_ob019L_100/1
  ACCSve_d_ACC_ISLCState/1 -> OMAP_Module/27(ACCSve_d_ACC_ISLCState)
  ACCSve_d_ACC_ISLCDriverRemind/1 -> OMAP_Module/28(ACCSve_d_ACC_ISLCDriverRemind)
  OMAP_Module/58(OMAPve_y_ADAS_ELKPopupMessage) -> OMAPve_y_ADAS_ELKPopupMessage/1
  OMAP_Module/59(OMAPve_y_ADAS_TurnLightsCommand) -> OMAPve_y_ADAS_TurnLightsCommand/1
  ESASve_y_ESA_State/1 -> OMAP_Module/114(ESASve_y_ESA_State)
  ESASve_g_ESA_SWA_CMD/1 -> OMAP_Module/115(ESASve_g_ESA_SWA_CMD)
  ESASve_g_EPS_Factor_Control/1 -> OMAP_Module/116(ESASve_g_EPS_Factor_Control)
  ESASve_y_ESA_FaultSt/1 -> OMAP_Module/117(ESASve_y_ESA_FaultSt)
  ESASve_y_ESARequest/1 -> OMAP_Module/118(ESASve_y_ESARequest)
  ESASve_y_ESATorqueReq/1 -> OMAP_Module/119(ESASve_y_ESATorqueReq)
  ESASve_y_LKAActivation/1 -> OMAP_Module/120(ESASve_y_LKAActivation)
  ACCSve_d_ACCMessagePrompt/1 -> OMAP_Module/26(ACCSve_d_ACCMessagePrompt)
  OMAP_Module/60(FDMMve_g_ob019H_100) -> FDMMve_g_ob019H_100/1
  IMAPve_d_L0_Q/1 -> OMAP_Module/121(IMAPve_d_L0_Q)
  IMAPve_d_R0_Q/1 -> OMAP_Module/122(IMAPve_d_R0_Q)

== system MIL4L3_SW6_V1_20220211/CarMaker/VehicleControl/SDFADataLog/Subsystem40/Subsystem ==
  Compare To Constant : simulink/Logic and Bit Operations/Compare To Constant  relop=>=  const=1  OutDataTypeStr=boolean
  Compare To Constant1 : simulink/Logic and Bit Operations/Compare To Constant  relop=>  const=0  OutDataTypeStr=boolean
  Const tar_id5 : Constant  Value=0
  Data Type Conversion : DataTypeConversion
  Digital Clock : DigitalClock  SampleTime=0.06
  Logical Operator : Logic  AllPortsSameDT=off  OutDataTypeStr=boolean
  Read CM Dict1 : CarMaker4SL/Read CM Dict  xname=Sensor.Object.Radar.relvTgt.dtct  xsync=off
  Read CM Dict7 : CarMaker4SL/Read CM Dict  xname=User.IO.Out.NumberOfObj  xsync=off
  Switch15 : Switch  Criteria=u2 > Threshold
  Radar_timestamp : Outport
  wires:
  Logical Operator/1 -> Switch15/2  "<dtct>"
  Digital Clock/1 -> Data Type Conversion/1
  Data Type Conversion/1 -> Switch15/1
  Switch15/1 -> Radar_timestamp/1  "Radar_timestamp"
  Const tar_id5/1 -> Switch15/3
  Read CM Dict7/1 -> Compare To Constant/1
  Compare To Constant/1 -> Logical Operator/2
  Read CM Dict1/1 -> Compare To Constant1/1
  Compare To Constant1/1 -> Logical Operator/1

== system MIL4L3_SW6_V1_20220211/CarMaker/VehicleControl/SDFADataLog/Subsystem40/Subsystem1 ==
  Compare To Constant : simulink/Logic and Bit Operations/Compare To Constant  relop=>=  const=2  OutDataTypeStr=boolean
  Compare To Constant1 : simulink/Logic and Bit Operations/Compare To Constant  relop=>  const=0  OutDataTypeStr=boolean
  Const tar_id5 : Constant  Value=0
  Data Type Conversion : DataTypeConversion
  Digital Clock : DigitalClock  SampleTime=0.06
  Logical Operator : Logic  AllPortsSameDT=off  OutDataTypeStr=boolean
  Read CM Dict1 : CarMaker4SL/Read CM Dict  xname=Sensor.Object.Radar.relvTgt.dtct  xsync=off
  Read CM Dict7 : CarMaker4SL/Read CM Dict  xname=User.IO.Out.NumberOfObj  xsync=off
  Switch15 : Switch  Criteria=u2 > Threshold
  Radar_timestamp : Outport
  wires:
  Compare To Constant1/1 -> Logical Operator/1
  Read CM Dict1/1 -> Compare To Constant1/1
  Compare To Constant/1 -> Logical Operator/2
  Read CM Dict7/1 -> Compare To Constant/1
  Const tar_id5/1 -> Switch15/3
  Switch15/1 -> Radar_timestamp/1  "Radar_timestamp"
  Data Type Conversion/1 -> Switch15/1
  Digital Clock/1 -> Data Type Conversion/1
  Logical Operator/1 -> Switch15/2  "<dtct>"

== system MIL4L3_SW6_V1_20220211/CarMaker/VehicleControl/SDFADataLog/Subsystem40/Subsystem2 ==
  Compare To Constant : simulink/Logic and Bit Operations/Compare To Constant  relop=>=  const=3  OutDataTypeStr=boolean
  Compare To Constant1 : simulink/Logic and Bit Operations/Compare To Constant  relop=>  const=0  OutDataTypeStr=boolean
  Const tar_id5 : Constant  Value=0
  Data Type Conversion : DataTypeConversion
  Digital Clock : DigitalClock  SampleTime=0.06
  Logical Operator : Logic  AllPortsSameDT=off  OutDataTypeStr=boolean
  Read CM Dict1 : CarMaker4SL/Read CM Dict  xname=Sensor.Object.Radar.relvTgt.dtct  xsync=off
  Read CM Dict7 : CarMaker4SL/Read CM Dict  xname=User.IO.Out.NumberOfObj  xsync=off
  Switch15 : Switch  Criteria=u2 > Threshold
  Radar_timestamp : Outport
  wires:
  Logical Operator/1 -> Switch15/2  "<dtct>"
  Digital Clock/1 -> Data Type Conversion/1
  Data Type Conversion/1 -> Switch15/1
  Switch15/1 -> Radar_timestamp/1  "Radar_timestamp"
  Const tar_id5/1 -> Switch15/3
  Read CM Dict7/1 -> Compare To Constant/1
  Compare To Constant/1 -> Logical Operator/2
  Read CM Dict1/1 -> Compare To Constant1/1
  Compare To Constant1/1 -> Logical Operator/1

== system MIL4L3_SW6_V1_20220211/CarMaker/VehicleControl/SDFADataLog/Subsystem40/Subsystem3 ==
  Compare To Constant : simulink/Logic and Bit Operations/Compare To Constant  relop=>=  const=4  OutDataTypeStr=boolean
  Compare To Constant1 : simulink/Logic and Bit Operations/Compare To Constant  relop=>  const=0  OutDataTypeStr=boolean
  Const tar_id5 : Constant  Value=0
  Data Type Conversion : DataTypeConversion
  Digital Clock : DigitalClock  SampleTime=0.06
  Logical Operator : Logic  AllPortsSameDT=off  OutDataTypeStr=boolean
  Read CM Dict1 : CarMaker4SL/Read CM Dict  xname=Sensor.Object.Radar.relvTgt.dtct  xsync=off
  Read CM Dict7 : CarMaker4SL/Read CM Dict  xname=User.IO.Out.NumberOfObj  xsync=off
  Switch15 : Switch  Criteria=u2 > Threshold
  Radar_timestamp : Outport
  wires:
  Compare To Constant1/1 -> Logical Operator/1
  Read CM Dict1/1 -> Compare To Constant1/1
  Compare To Constant/1 -> Logical Operator/2
  Read CM Dict7/1 -> Compare To Constant/1
  Const tar_id5/1 -> Switch15/3
  Switch15/1 -> Radar_timestamp/1  "Radar_timestamp"
  Data Type Conversion/1 -> Switch15/1
  Digital Clock/1 -> Data Type Conversion/1
  Logical Operator/1 -> Switch15/2  "<dtct>"

== system MIL4L3_SW6_V1_20220211/CarMaker/VehicleControl/SwitchForRealECU_ACC_Gas/PI Control/Subsystem1 ==
  -1 : Constant
  -2 : Constant
  -3 : Constant  Value=13.515
  -4 : Constant
  0 : Constant
  1 : Constant  Value=15.604
  2 : Constant  Value=11.1
  3 : Constant  Value=6.986
  4 : Constant  Value=4.737
  5 : Constant  Value=3.311
  6 : Constant  Value=2.356
  Multiport Switch : MultiPortSwitch  DataPortOrder=Specify indices  Inputs=9  DataPortIndices={0,1,2,3,4,5,6,7,8,-1}  DataPortForDefault=Additional data port
  Read CM Dict20 : CarMaker4SL/Read CM Dict  xname=PT.GearBox.GearNo  xsync=off
  TCU_AGB_position : Outport
  wires:
  -4/1 -> Multiport Switch/12
  -3/1 -> Multiport Switch/11
  Multiport Switch/1 -> TCU_AGB_position/1  "TCU_AGB_position"
  -2/1 -> Multiport Switch/10
  6/1 -> Multiport Switch/8
  1/1 -> Multiport Switch/3
  5/1 -> Multiport Switch/7
  2/1 -> Multiport Switch/4
  0/1 -> Multiport Switch/2
  -1/1 -> Multiport Switch/9
  4/1 -> Multiport Switch/6
  3/1 -> Multiport Switch/5
  Read CM Dict20/1 -> Multiport Switch/1

== system MIL4L3_SW6_V1_20220211/CarMaker/IPG Vehicle/CarAndTrailer/Forces/Tires/TireFL ==
  note: Insert your tire model here.
  Sync_In : Inport
  Load : Inport  Port=2
  vxtrans : Inport  Port=3
  vytrans : Inport  Port=4
  Rim_rotv : Inport  Port=5
  Rim_turnv : Inport  Port=6
  InclinAngle : Inport  Port=7
  muRoad : Inport  Port=8
  Ground{1..11} (11 alike) : Ground
  Terminator{,1..6,12} (8 alike) : Terminator
  Slp : Outport
  Alpha : Outport  Port=2
  TurnSlp : Outport  Port=3
  rBelt_eff : Outport  Port=4
  vBelt : Outport  Port=5
  LongFrc : Outport  Port=6
  SideFrc : Outport  Port=7
  LoadFrc : Outport  Port=8
  OverturnTrq : Outport  Port=9
  RollResist : Outport  Port=10
  AlignTrq : Outport  Port=11
  wires:
  Ground11/1 -> vBelt/1
  Ground10/1 -> rBelt_eff/1
  Ground9/1 -> TurnSlp/1
  Rim_turnv/1 -> Terminator6/1
  Sync_In/1 -> Terminator12/1
  Ground2/1 -> Alpha/1
  Ground3/1 -> LongFrc/1
  Ground4/1 -> SideFrc/1
  Ground5/1 -> OverturnTrq/1
  vxtrans/1 -> Terminator1/1
  vytrans/1 -> Terminator2/1
  Rim_rotv/1 -> Terminator3/1
  InclinAngle/1 -> Terminator4/1
  muRoad/1 -> Terminator5/1
  Load/1 -> Terminator/1
  Ground1/1 -> Slp/1
  Ground6/1 -> LoadFrc/1
  Ground7/1 -> RollResist/1
  Ground8/1 -> AlignTrq/1

== system MIL4L3_SW6_V1_20220211/CarMaker/IPG Vehicle/CarAndTrailer/Forces/Tires/TireFR ==
  note: Insert your tire model here.
  Sync_In : Inport
  Load : Inport  Port=2
  vxtrans : Inport  Port=3
  vytrans : Inport  Port=4
  Rim_rotv : Inport  Port=5
  Rim_turnv : Inport  Port=6
  InclinAngle : Inport  Port=7
  muRoad : Inport  Port=8
  Ground{1..11} (11 alike) : Ground
  Terminator{,1..6,12} (8 alike) : Terminator
  Slp : Outport
  Alpha : Outport  Port=2
  TurnSlp : Outport  Port=3
  rBelt_eff : Outport  Port=4
  vBelt : Outport  Port=5
  LongFrc : Outport  Port=6
  SideFrc : Outport  Port=7
  LoadFrc : Outport  Port=8
  OverturnTrq : Outport  Port=9
  RollResist : Outport  Port=10
  AlignTrq : Outport  Port=11
  wires:
  Ground11/1 -> vBelt/1
  Ground10/1 -> rBelt_eff/1
  Ground9/1 -> TurnSlp/1
  Rim_turnv/1 -> Terminator6/1
  Sync_In/1 -> Terminator12/1
  Ground2/1 -> Alpha/1
  Ground3/1 -> LongFrc/1
  Ground4/1 -> SideFrc/1
  Ground5/1 -> OverturnTrq/1
  vxtrans/1 -> Terminator1/1
  vytrans/1 -> Terminator2/1
  Rim_rotv/1 -> Terminator3/1
  InclinAngle/1 -> Terminator4/1
  muRoad/1 -> Terminator5/1
  Load/1 -> Terminator/1
  Ground1/1 -> Slp/1
  Ground6/1 -> LoadFrc/1
  Ground7/1 -> RollResist/1
  Ground8/1 -> AlignTrq/1

== system MIL4L3_SW6_V1_20220211/CarMaker/IPG Vehicle/CarAndTrailer/Forces/Tires/TireRL ==
  note: Insert your tire model here.
  Sync_In : Inport
  Load : Inport  Port=2
  vxtrans : Inport  Port=3
  vytrans : Inport  Port=4
  Rim_rotv : Inport  Port=5
  Rim_turnv : Inport  Port=6
  InclinAngle : Inport  Port=7
  muRoad : Inport  Port=8
  Ground{1..11} (11 alike) : Ground
  Terminator{,1..6,12} (8 alike) : Terminator
  Slp : Outport
  Alpha : Outport  Port=2
  TurnSlp : Outport  Port=3
  rBelt_eff : Outport  Port=4
  vBelt : Outport  Port=5
  LongFrc : Outport  Port=6
  SideFrc : Outport  Port=7
  LoadFrc : Outport  Port=8
  OverturnTrq : Outport  Port=9
  RollResist : Outport  Port=10
  AlignTrq : Outport  Port=11
  wires:
  Ground11/1 -> vBelt/1
  Ground10/1 -> rBelt_eff/1
  Ground9/1 -> TurnSlp/1
  Rim_turnv/1 -> Terminator6/1
  Sync_In/1 -> Terminator12/1
  Ground2/1 -> Alpha/1
  Ground3/1 -> LongFrc/1
  Ground4/1 -> SideFrc/1
  Ground5/1 -> OverturnTrq/1
  vxtrans/1 -> Terminator1/1
  vytrans/1 -> Terminator2/1
  Rim_rotv/1 -> Terminator3/1
  InclinAngle/1 -> Terminator4/1
  muRoad/1 -> Terminator5/1
  Load/1 -> Terminator/1
  Ground1/1 -> Slp/1
  Ground6/1 -> LoadFrc/1
  Ground7/1 -> RollResist/1
  Ground8/1 -> AlignTrq/1

== system MIL4L3_SW6_V1_20220211/CarMaker/IPG Vehicle/CarAndTrailer/Forces/Tires/TireRR ==
  note: Insert your tire model here.
  Sync_In : Inport
  Load : Inport  Port=2
  vxtrans : Inport  Port=3
  vytrans : Inport  Port=4
  Rim_rotv : Inport  Port=5
  Rim_turnv : Inport  Port=6
  InclinAngle : Inport  Port=7
  muRoad : Inport  Port=8
  Ground{1..11} (11 alike) : Ground
  Terminator{,1..6,12} (8 alike) : Terminator
  Slp : Outport
  Alpha : Outport  Port=2
  TurnSlp : Outport  Port=3
  rBelt_eff : Outport  Port=4
  vBelt : Outport  Port=5
  LongFrc : Outport  Port=6
  SideFrc : Outport  Port=7
  LoadFrc : Outport  Port=8
  OverturnTrq : Outport  Port=9
  RollResist : Outport  Port=10
  AlignTrq : Outport  Port=11
  wires:
  Ground11/1 -> vBelt/1
  Ground10/1 -> rBelt_eff/1
  Ground9/1 -> TurnSlp/1
  Rim_turnv/1 -> Terminator6/1
  Sync_In/1 -> Terminator12/1
  Ground2/1 -> Alpha/1
  Ground3/1 -> LongFrc/1
  Ground4/1 -> SideFrc/1
  Ground5/1 -> OverturnTrq/1
  vxtrans/1 -> Terminator1/1
  vytrans/1 -> Terminator2/1
  Rim_rotv/1 -> Terminator3/1
  InclinAngle/1 -> Terminator4/1
  muRoad/1 -> Terminator5/1
  Load/1 -> Terminator/1
  Ground1/1 -> Slp/1
  Ground6/1 -> LoadFrc/1
  Ground7/1 -> RollResist/1
  Ground8/1 -> AlignTrq/1
